simulink model "PIDTestSim"  (R2016b)
settings: Solver=VariableStepAuto  StartTime=0.0  StopTime=100  RelTol=1e-3
undefined symbols (not defined in the file or in its folder): DrawPlane, GetForces, P, Sensor
libraries: simulink x5
settings Model: Creator=CFRPG  LastModifiedBy=CFRPG

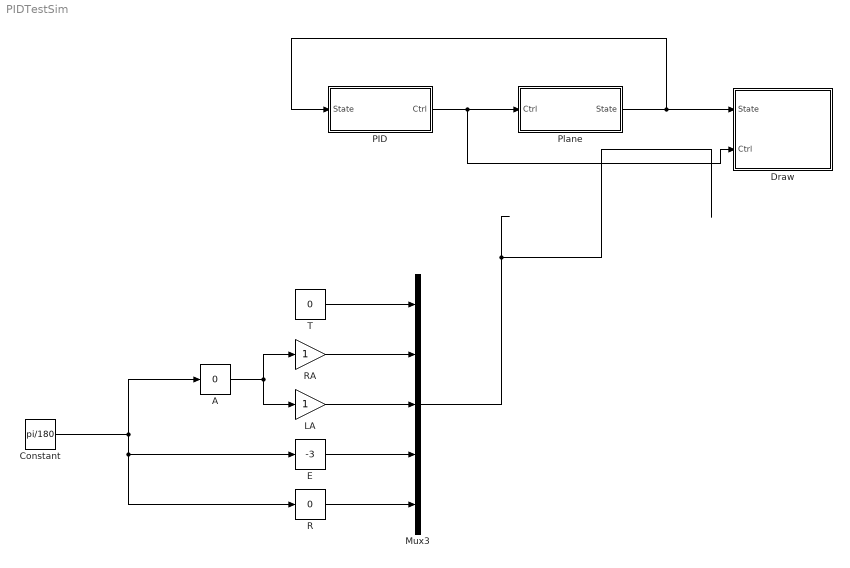
== system PIDTestSim ==
  A : simulink/Math Operations/Slider Gain  low=-360  gain=0  high=360
  Constant : Constant  Value=pi/180
  Draw : Subsystem
  E : simulink/Math Operations/Slider Gain  low=-360  gain=-3  high=360
  LA : Gain
  Mux3 : Mux  Inputs=5
  PID : Subsystem
  Plane : Subsystem
  R : simulink/Math Operations/Slider Gain  low=-360  gain=0  high=360
  RA : Gain
  T : Constant  Value=0
  wires:
  Plane/1(State) -> PID/1(State), Draw/1(State)
  R/1 -> Mux3/5
  E/1 -> Mux3/4
  T/1 -> Mux3/1
  RA/1 -> Mux3/2
  LA/1 -> Mux3/3
  A/1 -> RA/1, LA/1
  Constant/1 -> A/1, E/1, R/1
  Mux3/1 -> ?
  PID/1(Ctrl) -> Plane/1(Ctrl), Draw/2(Ctrl)

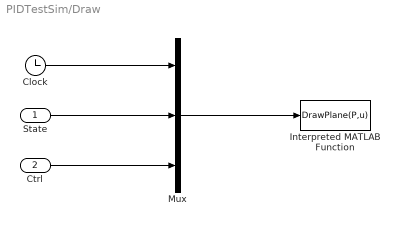
== system PIDTestSim/Draw ==
  State : Inport
  Ctrl : Inport  Port=2
  Clock : Clock
  Interpreted MATLAB Function : MATLABFcn  MATLABFcn=DrawPlane(P,u)  OutputDimensions=0
  Mux : Mux  Inputs=3
  wires:
  State/1 -> Mux/2
  Clock/1 -> Mux/1
  Ctrl/1 -> Mux/3
  Mux/1 -> Interpreted MATLAB Function/1

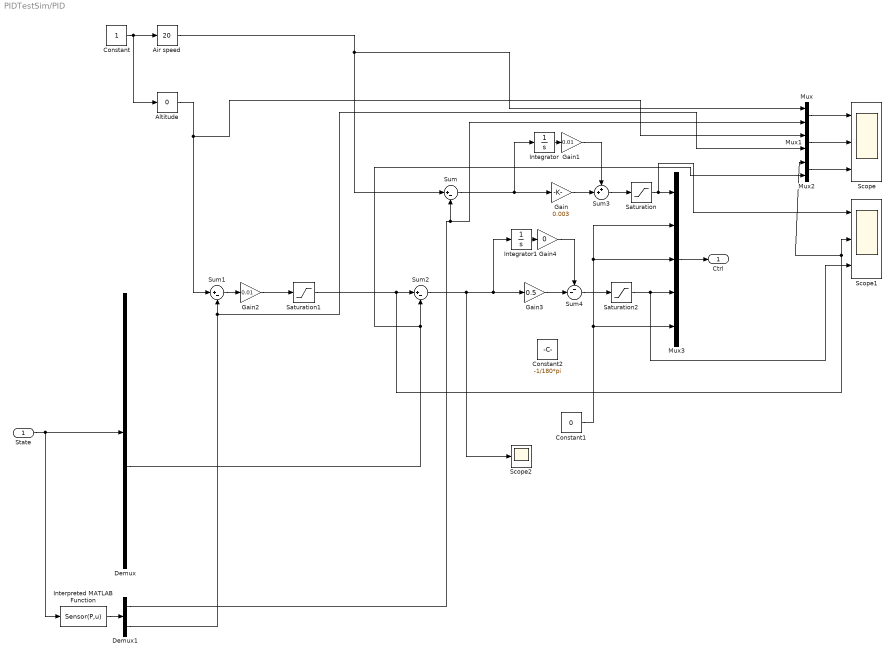
== system PIDTestSim/PID ==
  State : Inport
  Air speed : simulink/Math Operations/Slider Gain  low=0  gain=20  high=50
  Altitude : simulink/Math Operations/Slider Gain  low=-100  gain=0  high=100
  Constant : Constant
  Constant1 : Constant  Value=0
  Constant2 : Constant  Value=-1/180*pi
  Demux : Demux  Outputs=12
  Demux1 : Demux  Outputs=2
  Gain : Gain  Gain=0.003
  Gain1 : Gain  Gain=0.01
  Gain2 : Gain  Gain=0.01
  Gain3 : Gain  Gain=0.5
  Gain4 : Gain  Gain=0
  Integrator : Integrator
  Integrator1 : Integrator
  Interpreted MATLAB Function : MATLABFcn  MATLABFcn=Sensor(P,u)
  Mux : Mux  Inputs=2
  Mux1 : Mux  Inputs=2
  Mux2 : Mux  Inputs=2
  Mux3 : Mux  Inputs=5
  Saturation : Saturate  UpperLimit=1  LowerLimit=0
  Saturation1 : Saturate  UpperLimit=pi/9  LowerLimit=-pi/9
  Saturation2 : Saturate  UpperLimit=pi/9  LowerLimit=-pi/9
  Scope : Scope  NumInputPorts=3
  Scope1 : Scope  NumInputPorts=3
  Scope2 : Scope
  Sum : Sum  Inputs=|+-
  Sum1 : Sum  Inputs=|+-
  Sum2 : Sum  Inputs=|+-
  Sum3 : Sum  Inputs=++|
  Sum4 : Sum  Inputs=--|
  Ctrl : Outport
  wires:
  State/1 -> Interpreted MATLAB Function/1, Demux/1
  Mux3/1 -> Ctrl/1
  Interpreted MATLAB Function/1 -> Demux1/1
  Sum/1 -> Integrator/1, Gain/1
  Saturation/1 -> Scope1/1, Mux3/1
  Constant/1 -> Altitude/1, Air speed/1
  Air speed/1 -> Mux/1, Sum/1
  Demux1/1 -> Mux/2, Sum/2
  Altitude/1 -> Mux1/1, Sum1/1
  Demux1/2 -> Mux1/2, Sum1/2
  Sum1/1 -> Gain2/1
  Demux/8 -> Mux2/2, Sum2/2
  Saturation2/1 -> Mux3/4, Scope1/3
  Sum2/1 -> Scope2/1, Integrator1/1, Gain3/1
  Constant1/1 -> Mux3/5, Mux3/2, Mux3/3
  Gain2/1 -> Saturation1/1
  Gain/1 -> Sum3/2
  Gain3/1 -> Sum4/2
  Sum3/1 -> Saturation/1
  Integrator/1 -> Gain1/1
  Gain1/1 -> Sum3/1
  Mux/1 -> Scope/1
  Mux1/1 -> Scope/2
  Mux2/1 -> Scope/3
  Sum4/1 -> Saturation2/1
  Integrator1/1 -> Gain4/1
  Gain4/1 -> Sum4/1
  Saturation1/1 -> Mux2/1, Scope1/2, Sum2/1

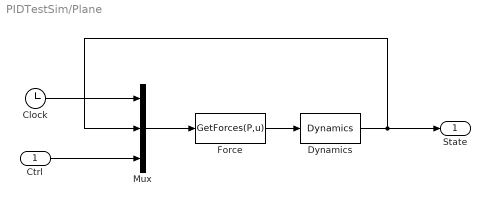
== system PIDTestSim/Plane ==
  Ctrl : Inport
  Clock : Clock
  Dynamics : S-Function  FunctionName=Dynamics  Parameters=P  SFunctionDeploymentMode=off  EnableBusSupport=off
  Force : MATLABFcn  MATLABFcn=GetForces(P,u)
  Mux : Mux  Inputs=3
  State : Outport
  wires:
  Ctrl/1 -> Mux/3
  Dynamics/1 -> Mux/2, State/1
  Force/1 -> Dynamics/1
  Mux/1 -> Force/1
  Clock/1 -> Mux/1
